simulink model "TNC1"  (R2021b)
settings: Solver=FixedStepDiscrete  StartTime=0.0  StopTime=1  FixedStep=0.001  RelTol=1e-3
settings Model: Creator=10373  LastModifiedBy=黄艳龙
settings OptimizationCC: DefaultParameterBehavior=Inlined  EnhancedBackFolding=on  PassReuseOutputArgsAs=Individual arguments  ZeroExternalMemoryAtStartup=off  ZeroInternalMemoryAtStartup=off  NoFixptDivByZeroProtection=on  EfficientFloat2IntCast=on  OptimizeBlockOrder=speed  DifferentSizesBufferReuse=on  OptimizationCustomize=off  EfficientTunableParamExpr=on
settings DebuggingCC: ParameterTunabilityLossMsg=error
settings HardwareCC: ProdBitPerPointer=32  ProdBitPerSizeT=32  ProdBitPerPtrDiffT=32  ProdLargestAtomicInteger=Long  ProdLargestAtomicFloat=Double  ProdWordSize=32  ProdLongLongMode=on  ProdHWDeviceType=NXP->Cortex-M3
settings SFSimCC: MATLABDynamicMemAlloc=off
settings RTWCC: Description=Embedded Coder  SystemTargetFile=ert.tlc  GenCodeOnly=on  TemplateMakefile=ert_default_tmf  GenerateReport=on  LaunchReport=on
settings CodeAppCC: ForceParamTrailComments=on  IgnoreCustomStorageClasses=off  MaxIdLength=256  OperatorAnnotations=on  SimulinkDataObjDesc=on  SFDataObjDesc=on  InsertBlockDesc=on
settings ERTTargetCC: TargetLangStandard=C99 (ISO)  SuppressErrorStatus=on  SupportNonFinite=off  InlinedParameterPlacement=NonHierarchical  ERTCustomFileTemplate=example_file_process.tlc

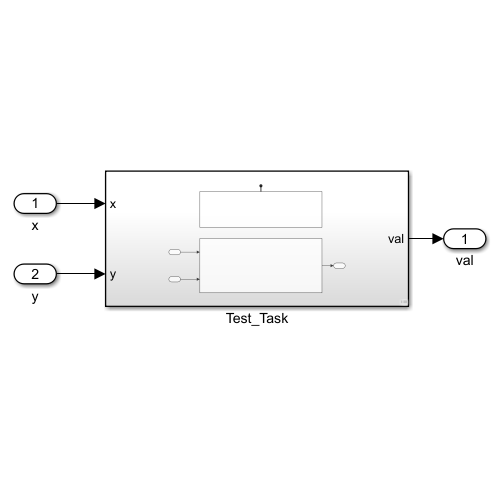
[thumbnail: Simulink's stored preview of the top-level diagram]
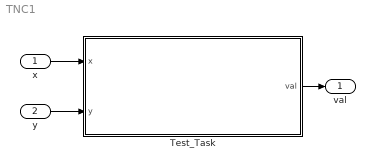
== system TNC1 ==
  x : Inport  OutDataTypeStr=uint16
  y : Inport  Port=2  OutDataTypeStr=uint16
  Test_Task : Subsystem
  val : Outport  OutDataTypeStr=uint16
  wires:
  Test_Task/1(val) -> val/1
  x/1 -> Test_Task/1(x)
  y/1 -> Test_Task/2(y)

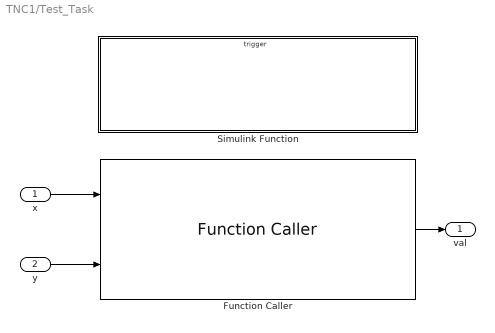
== system TNC1/Test_Task ==
  x : Inport  OutDataTypeStr=uint16
  y : Inport  Port=2  OutDataTypeStr=uint16
  Function Caller : FunctionCaller  FunctionPrototype=val = add(x,y)  InputArgumentSpecifications=uint16(1),uint16(1)  OutputArgumentSpecifications=uint16(1)
  Simulink Function : Subsystem  TreatAsAtomicUnit=on
  val : Outport  OutDataTypeStr=uint16
  wires:
  x/1 -> Function Caller/1
  y/1 -> Function Caller/2
  Function Caller/1 -> val/1

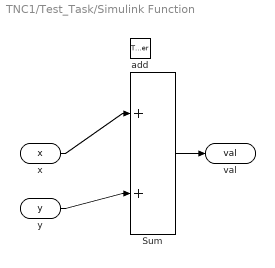
== system TNC1/Test_Task/Simulink Function ==
  add : TriggerPort  TriggerType=function-call  IsSimulinkFunction=on  FunctionName=add  FunctionVisibility=scoped  VariantControl=(inherit)
  Sum : Sum  Inputs=|++
  x : ArgIn  DisableCoverage=on  OutDataTypeStr=uint16  ArgumentName=x
  y : ArgIn  Port=2  OutDataTypeStr=uint16  ArgumentName=y
  val : ArgOut  OutDataTypeStr=uint16  ArgumentName=val
  wires:
  x/1 -> Sum/1
  y/1 -> Sum/2
  Sum/1 -> val/1
